simulink model "untitled"  (R2020b)
settings: Solver=VariableStepAuto  StartTime=0.0  StopTime=500  FixedStep=0.000001  MaxStep=1e-4  RelTol=1e-3  EnableMultiTasking=on
libraries: dsparch4 x4, dspsrcs4 x4, simulink x2, dspfdesign x2
(part 1 of 4)
settings Model: Creator=LYX  LastModifiedBy=LYX

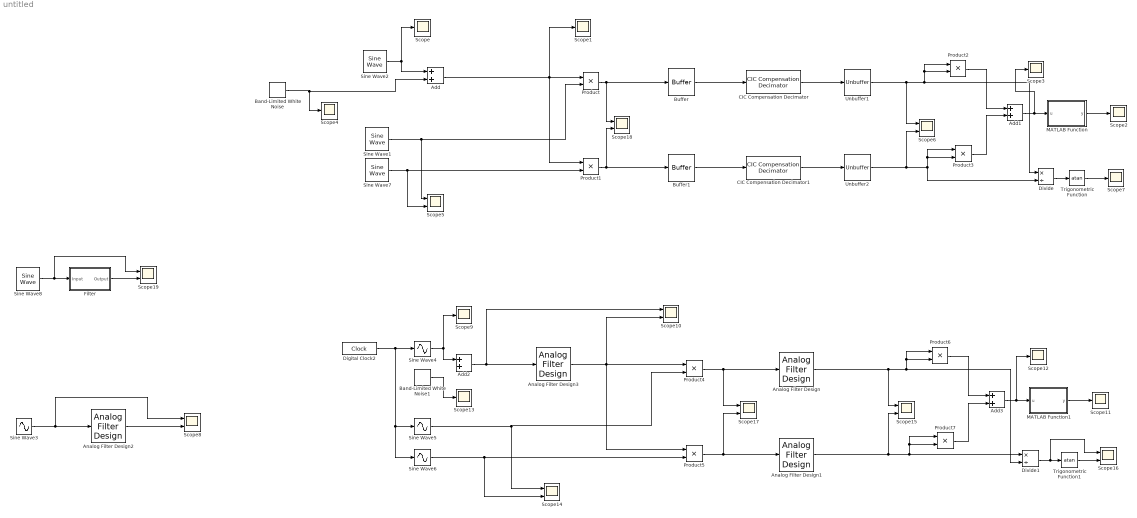
== system untitled ==
  Add{,1..3} (4 alike) : Sum
  Analog Filter Design : dsparch4/Analog Filter Design  method=Butterworth  filttype=Lowpass  N=8  Wlo=0.1  Whi=80  Rp=2  Rs=40
  Analog Filter Design1 : dsparch4/Analog Filter Design  method=Butterworth  filttype=Lowpass  N=8  Wlo=0.1  Whi=80  Rp=2  Rs=40
  Analog Filter Design2 : dsparch4/Analog Filter Design  method=Butterworth  filttype=Bandpass  N=2  Wlo=20*pi  Whi=60*pi  Rp=2  Rs=40
  Analog Filter Design3 : dsparch4/Analog Filter Design  method=Butterworth  filttype=Bandpass  N=8  Wlo=30*pi  Whi=50*pi  Rp=2  Rs=40
  Band-Limited White Noise : simulink/Sources/Band-Limited White Noise  Cov=[0.00001*0.00001*0.01]  Ts=0.1  seed=[23341]
  Band-Limited White Noise1 : simulink/Sources/Band-Limited White Noise  Cov=[0.00001*0.00001*0.01]  Ts=0.1  seed=[23341]
  Buffer : Buffer  N=8  OutputFrames=off
  Buffer1 : Buffer  N=8  OutputFrames=off
  CIC Compensation Decimator : dspfdesign/CIC Compensation Decimator  CICRateChangeFactor=4  CICNumSections=5  CICDifferentialDelay=1  DecimationFactor=4  DesignForMinimumOrder=on  FilterOrder=12  PassbandFrequency=1  StopbandFrequency=6  PassbandRipple=0.1  StopbandAttenuation=60  InheritSampleRate=on  SampleRate=1200000  SimulateUsing=Code generation  roundingMode=Floor  coeffsDataTypeStr=fixdt(1,16)
      settings: SourceProductBaseCode=DS
  CIC Compensation Decimator1 : dspfdesign/CIC Compensation Decimator  CICRateChangeFactor=4  CICNumSections=5  CICDifferentialDelay=1  DecimationFactor=4  DesignForMinimumOrder=on  FilterOrder=12  PassbandFrequency=1  StopbandFrequency=6  PassbandRipple=0.1  StopbandAttenuation=60  InheritSampleRate=on  SampleRate=1200000  SimulateUsing=Code generation  roundingMode=Floor  coeffsDataTypeStr=fixdt(1,16)
      settings: SourceProductBaseCode=DS
  Digital Clock2 : DigitalClock  SampleTime=0.001
  Divide : Product  Inputs=*/
  Divide1 : Product  Inputs=*/
  Filter : Subsystem  Tag=FilterWizardSubSystem
      settings: ErrorFcn=dspFilterRealizedInBasicElemsAlgLoopErrFcnCallback
  MATLAB Function : MATLAB Function  TreatAsAtomicUnit=on
  MATLAB Function1 : MATLAB Function  TreatAsAtomicUnit=on
  Product{,1..7} (8 alike) : Product
  Scope{,1..4,7,9,11..13} (10 alike) : Scope
  Scope{5..6,8,10,14..19} (10 alike) : Scope  NumInputPorts=2
  Sine Wave1 : dspsrcs4/Sine Wave  Amplitude=1  Frequency=20  Phase=0  SampleMode=Discrete  OutComplex=Real  CompMethod=Trigonometric fcn  TableSize=Speed  SampleTime=1/1000  SamplesPerFrame=1  ResetState=Restart at time zero  OutputFrames=off  dataType=double  wordLen=16  udDataType=sfix(16)  fracBitsMode=Best precision  numFracBits=15  OutDataTypeStr=double  LastOutDataTypeStr=double
  Sine Wave2 : dspsrcs4/Sine Wave  Amplitude=0.05  Frequency=19.5  Phase=0  SampleMode=Discrete  OutComplex=Real  CompMethod=Trigonometric fcn  TableSize=Speed  SampleTime=1/1000  SamplesPerFrame=1  ResetState=Restart at time zero  OutputFrames=off  dataType=double  wordLen=16  udDataType=sfix(16)  fracBitsMode=Best precision  numFracBits=15  OutDataTypeStr=double  LastOutDataTypeStr=double
  Sine Wave3 : Sin  Amplitude=2  Frequency=40*pi  Samples=50  SampleTime=0
  Sine Wave4 : Sin  SineType=Sample based  TimeSource=Use external signal  Amplitude=0.00001  Frequency=40*pi  Samples=50  SampleTime=0.001
  Sine Wave5 : Sin  SineType=Sample based  TimeSource=Use external signal  Frequency=40*pi  Samples=50  SampleTime=0.001
  Sine Wave6 : Sin  SineType=Sample based  TimeSource=Use external signal  Frequency=40*pi  Phase=pi/2  Samples=50  SampleTime=0.001  Offset=12.5
  Sine Wave7 : dspsrcs4/Sine Wave  Amplitude=1  Frequency=20  Phase=pi/2  SampleMode=Discrete  OutComplex=Real  CompMethod=Trigonometric fcn  TableSize=Speed  SampleTime=1/1000  SamplesPerFrame=1  ResetState=Restart at time zero  OutputFrames=off  dataType=double  wordLen=16  udDataType=sfix(16)  fracBitsMode=Best precision  numFracBits=15  OutDataTypeStr=double  LastOutDataTypeStr=double
  Sine Wave8 : dspsrcs4/Sine Wave  Amplitude=2  Frequency=20  Phase=0  SampleMode=Discrete  OutComplex=Real  CompMethod=Trigonometric fcn  TableSize=Speed  SampleTime=1/1000  SamplesPerFrame=1  ResetState=Restart at time zero  OutputFrames=off  dataType=double  wordLen=16  udDataType=sfix(16)  fracBitsMode=Best precision  numFracBits=15  OutDataTypeStr=double  LastOutDataTypeStr=double
  Trigonometric Function : Trigonometry  Operator=atan
  Trigonometric Function1 : Trigonometry  Operator=atan
  Unbuffer1 : Unbuffer
  Unbuffer2 : Unbuffer
  wires:
  Sine Wave2/1 -> Add/1, Scope/1
  Band-Limited White Noise/1 -> Add/2, Scope4/1
  Sine Wave1/1 -> Scope5/1, Product/2
  Sine Wave7/1 -> Scope5/2, Product1/2
  Product2/1 -> Add1/1
  Product3/1 -> Add1/2
  Add1/1 -> Scope3/1, MATLAB Function/1(u)
  MATLAB Function/1(y) -> Scope2/1
  Divide/1 -> Trigonometric Function/1
  Trigonometric Function/1 -> Scope7/1
  Unbuffer1/1 -> Scope6/1, Divide/1, Product2/2, Product2/1
  Unbuffer2/1 -> Scope6/2, Divide/2, Product3/2, Product3/1
  Analog Filter Design1/1 -> Scope15/2, Product7/2, Product7/1, Divide1/1
  Digital Clock2/1 -> Sine Wave4/1, Sine Wave5/1, Sine Wave6/1
  Sine Wave4/1 -> Add2/1, Scope9/1
  Trigonometric Function1/1 -> Scope16/2
  Divide1/1 -> Scope16/1, Trigonometric Function1/1
  Analog Filter Design/1 -> Scope15/1, Divide1/2, Product6/2, Product6/1
  Band-Limited White Noise1/1 -> Scope13/1
  Product6/1 -> Add3/1
  Add3/1 -> Scope12/1, MATLAB Function1/1(u)
  Sine Wave5/1 -> Scope14/1, Product4/2
  Product7/1 -> Add3/2
  MATLAB Function1/1(y) -> Scope11/1
  Sine Wave6/1 -> Scope14/2, Product5/2
  CIC Compensation Decimator/1 -> Unbuffer1/1
  CIC Compensation Decimator1/1 -> Unbuffer2/1
  Product/1 -> Buffer/1, Scope18/1
  Product1/1 -> Buffer1/1, Scope18/2
  Buffer/1 -> CIC Compensation Decimator/1
  Buffer1/1 -> CIC Compensation Decimator1/1
  Product5/1 -> Analog Filter Design1/1, Scope17/2
  Product4/1 -> Scope17/1, Analog Filter Design/1
  Sine Wave3/1 -> Scope8/1, Analog Filter Design2/1
  Analog Filter Design2/1 -> Scope8/2
  Add2/1 -> Analog Filter Design3/1, Scope10/1
  Add/1 -> Product1/1, Scope1/1, Product/1
  Sine Wave8/1 -> Filter/1(Input), Scope19/1
  Filter/1(Output) -> Scope19/2
  Analog Filter Design3/1 -> Product5/1, Scope10/2, Product4/1
